simulink model "reverserotor"  (Simulink 10.0)
settings: Solver=ode23t  StartTime=0.0  StopTime=2  RelTol=1e-3  EnableMultiTasking=on
settings Model: Creator=lenovo  LastModifiedBy=asuresh4
settings DataIOCC: LimitDataPoints=on  SignalLoggingSaveFormat=ModelDataLogs
settings OptimizationCC: ExpressionDepthLimit=2147483647
settings DebuggingCC: SolverPrmCheckMsg=warning  FcnCallInpInsideContextMsg=warning  StateNameClashWarn=warning
settings ConfigComp: CovExternalEMLEnable=off

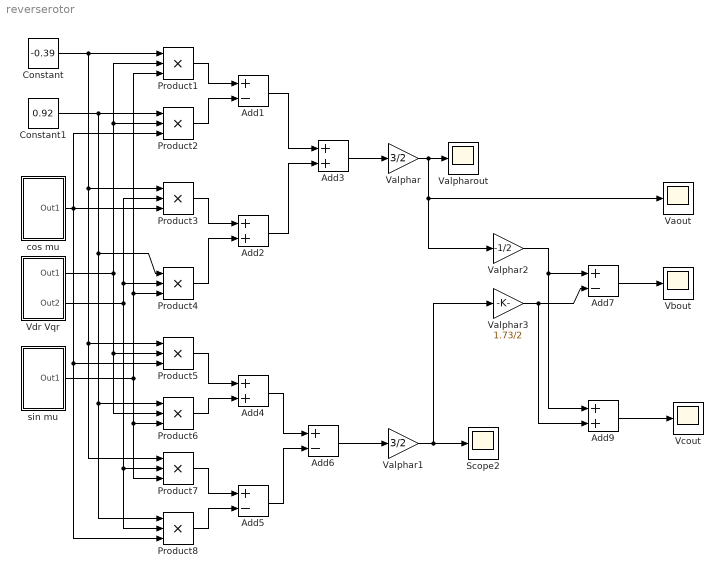
== system reverserotor ==
  Add{1,5..7} (4 alike) : Sum  Inputs=+-
  Add{2..4,9} (4 alike) : Sum
  Constant : Constant  Value=-0.39
  Constant1 : Constant  Value=0.92
  Product{1..8} (8 alike) : Product  Inputs=3  RndMeth=Zero
  Scope2 : Scope
  Valphar : Gain  Gain=3/2
  Valphar1 : Gain  Gain=3/2
  Valphar2 : Gain  Gain=-1/2
  Valphar3 : Gain  Gain=1.73/2
  Valpharout : Scope
  Vaout : Scope
  Vbout : Scope
  Vcout : Scope
  Vdr Vqr : Subsystem
  cos mu : Subsystem
  sin mu : Subsystem
  wires:
  Constant/1 -> Product1/1, Product3/1, Product5/1, Product7/1
  Vdr Vqr/1(Out1) -> Product1/2, Product2/2, Product5/2, Product6/2
  sin mu/1(Out1) -> Product1/3, Product4/3, Product6/3, Product7/3
  Constant1/1 -> Product2/1, Product4/1, Product6/1, Product8/1
  cos mu/1(Out1) -> Product3/3, Product2/3, Product5/3, Product8/3
  Product1/1 -> Add1/1
  Product2/1 -> Add1/2
  Vdr Vqr/2(Out2) -> Product3/2, Product4/2, Product7/2, Product8/2
  Product3/1 -> Add2/1
  Product4/1 -> Add2/2
  Add1/1 -> Add3/1
  Add2/1 -> Add3/2
  Add3/1 -> Valphar/1
  Valphar/1 -> Vaout/1, Valphar2/1, Valpharout/1
  Valphar1/1 -> Scope2/1, Valphar3/1
  Add6/1 -> Valphar1/1
  Add4/1 -> Add6/1
  Add5/1 -> Add6/2
  Product5/1 -> Add4/1
  Product6/1 -> Add4/2
  Product7/1 -> Add5/1
  Product8/1 -> Add5/2
  Add7/1 -> Vbout/1
  Valphar3/1 -> Add7/2, Add9/2
  Valphar2/1 -> Add7/1, Add9/1
  Add9/1 -> Vcout/1

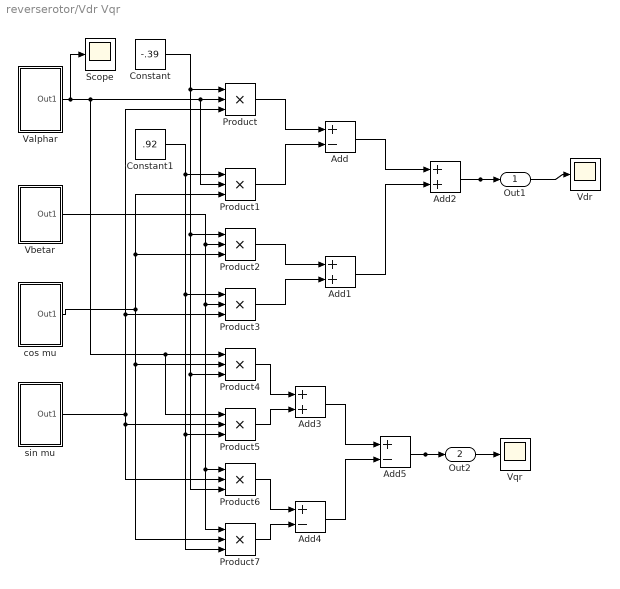
== system reverserotor/Vdr Vqr ==
  Add : Sum  Inputs=+-
  Add1 : Sum
  Add2 : Sum
  Add3 : Sum
  Add4 : Sum  Inputs=+-
  Add5 : Sum  Inputs=+-
  Constant : Constant  Value=-.39
  Constant1 : Constant  Value=.92
  Product{,1..7} (8 alike) : Product  Inputs=3  RndMeth=Zero
  Scope : Scope
  Valphar : Subsystem
  Vbetar : Subsystem
  Vdr : Scope
  Vqr : Scope
  cos mu : Subsystem
  sin mu : Subsystem
  Out1 : Outport
  Out2 : Outport  Port=2
  wires:
  Constant/1 -> Product/1, Product2/1, Product4/3, Product6/3
  sin mu/1(Out1) -> Product/3, Product3/3, Product5/2, Product6/2
  Valphar/1(Out1) -> Product/2, Product1/2, Product4/1, Product5/1, Scope/1
  Constant1/1 -> Product1/1, Product3/1, Product5/3, Product7/3
  cos mu/1(Out1) -> Product1/3, Product2/3, Product4/2, Product7/2
  Product/1 -> Add/1
  Product1/1 -> Add/2
  Vbetar/1(Out1) -> Product2/2, Product3/2, Product6/1, Product7/1
  Product2/1 -> Add1/1
  Product3/1 -> Add1/2
  Add/1 -> Add2/1
  Add1/1 -> Add2/2
  Add2/1 -> Vdr/1, Out1/1
  Product4/1 -> Add3/1
  Product5/1 -> Add3/2
  Product6/1 -> Add4/1
  Product7/1 -> Add4/2
  Add3/1 -> Add5/1
  Add4/1 -> Add5/2
  Add5/1 -> Vqr/1, Out2/1

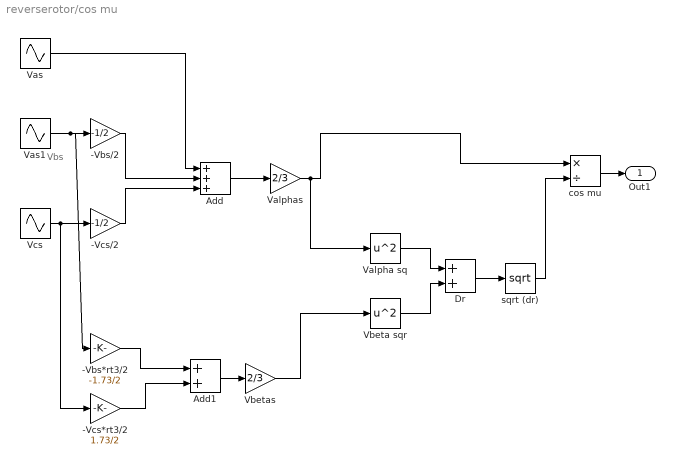
== system reverserotor/cos mu ==
  note: Vbs
  -Vbs*rt3/2 : Gain  Gain=-1.73/2
  -Vbs/2 : Gain  Gain=-1/2
  -Vcs*rt3/2 : Gain  Gain=1.73/2
  -Vcs/2 : Gain  Gain=-1/2
  Add : Sum  Inputs=+++
  Add1 : Sum
  Dr : Sum
  Valpha sq : Math  Operator=square  SaturateOnIntegerOverflow=on
  Valphas : Gain  Gain=2/3
  Vas : Sin  Amplitude=230  Frequency=314  SampleTime=0
  Vas1 : Sin  Amplitude=230  Frequency=314  Phase=-2.09  SampleTime=0
  Vbeta sqr : Math  Operator=square  SaturateOnIntegerOverflow=on
  Vbetas : Gain  Gain=2/3
  Vcs : Sin  Amplitude=230  Frequency=314  Phase=-4.18  SampleTime=0
  cos mu : Product  Inputs=*/
  sqrt (dr) : Math  Operator=sqrt  SaturateOnIntegerOverflow=on
  Out1 : Outport
  wires:
  Vas1/1 -> -Vbs/2/1, -Vbs*rt3/2/1
  Vcs/1 -> -Vcs/2/1, -Vcs*rt3/2/1
  Vas/1 -> Add/1
  -Vbs/2/1 -> Add/2
  -Vcs/2/1 -> Add/3
  Add/1 -> Valphas/1
  -Vbs*rt3/2/1 -> Add1/1
  -Vcs*rt3/2/1 -> Add1/2
  Add1/1 -> Vbetas/1
  Valphas/1 -> Valpha sq/1, cos mu/1
  Vbetas/1 -> Vbeta sqr/1
  Valpha sq/1 -> Dr/1
  Vbeta sqr/1 -> Dr/2
  Dr/1 -> sqrt (dr)/1
  sqrt (dr)/1 -> cos mu/2
  cos mu/1 -> Out1/1

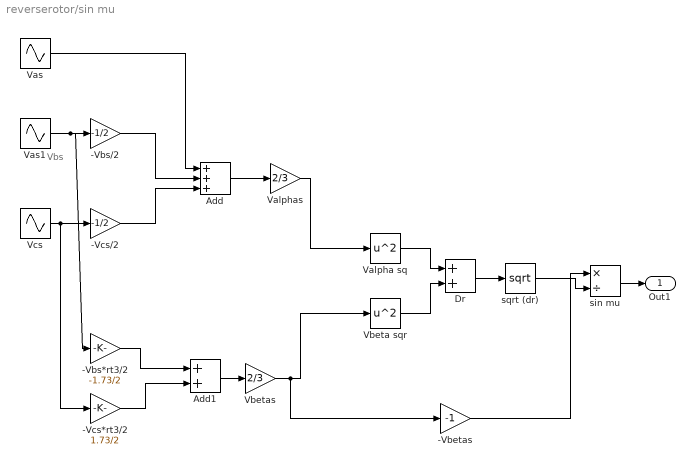
== system reverserotor/sin mu ==
  note: Vbs
  "-Vbetas " : Gain  Gain=-1
  -Vbs*rt3/2 : Gain  Gain=-1.73/2
  -Vbs/2 : Gain  Gain=-1/2
  -Vcs*rt3/2 : Gain  Gain=1.73/2
  -Vcs/2 : Gain  Gain=-1/2
  Add : Sum  Inputs=+++
  Add1 : Sum
  Dr : Sum
  Valpha sq : Math  Operator=square  SaturateOnIntegerOverflow=on
  Valphas : Gain  Gain=2/3
  Vas : Sin  Amplitude=230  Frequency=314  SampleTime=0
  Vas1 : Sin  Amplitude=230  Frequency=314  Phase=-2.09  SampleTime=0
  Vbeta sqr : Math  Operator=square  SaturateOnIntegerOverflow=on
  Vbetas : Gain  Gain=2/3
  Vcs : Sin  Amplitude=230  Frequency=314  Phase=-4.18  SampleTime=0
  sin mu : Product  Inputs=*/
  sqrt (dr) : Math  Operator=sqrt  SaturateOnIntegerOverflow=on
  Out1 : Outport
  wires:
  Vas1/1 -> -Vbs/2/1, -Vbs*rt3/2/1
  Vcs/1 -> -Vcs/2/1, -Vcs*rt3/2/1
  Vas/1 -> Add/1
  -Vbs/2/1 -> Add/2
  -Vcs/2/1 -> Add/3
  Add/1 -> Valphas/1
  -Vbs*rt3/2/1 -> Add1/1
  -Vcs*rt3/2/1 -> Add1/2
  Add1/1 -> Vbetas/1
  Valphas/1 -> Valpha sq/1
  Vbetas/1 -> "-Vbetas "/1, Vbeta sqr/1
  Valpha sq/1 -> Dr/1
  Vbeta sqr/1 -> Dr/2
  Dr/1 -> sqrt (dr)/1
  "-Vbetas "/1 -> sin mu/1
  sqrt (dr)/1 -> sin mu/2
  sin mu/1 -> Out1/1

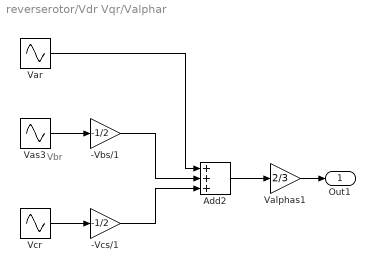
== system reverserotor/Vdr Vqr/Valphar ==
  note: Vbr
  -Vbs/1 : Gain  Gain=-1/2
  -Vcs/1 : Gain  Gain=-1/2
  Add2 : Sum  Inputs=+++
  Valphas1 : Gain  Gain=2/3
  Var : Sin  Amplitude=69  Frequency=314  SampleTime=0
  Vas3 : Sin  Amplitude=69  Frequency=314  Phase=-2.09  SampleTime=0
  Vcr : Sin  Amplitude=69  Frequency=314  Phase=-4.18  SampleTime=0
  Out1 : Outport
  wires:
  Vas3/1 -> -Vbs/1/1
  Vcr/1 -> -Vcs/1/1
  Var/1 -> Add2/1
  -Vbs/1/1 -> Add2/2
  -Vcs/1/1 -> Add2/3
  Add2/1 -> Valphas1/1
  Valphas1/1 -> Out1/1

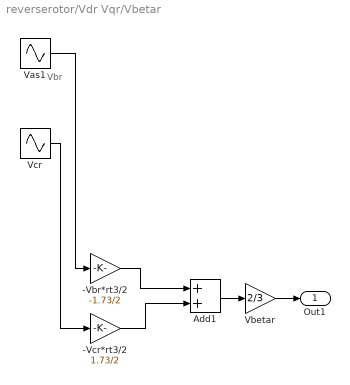
== system reverserotor/Vdr Vqr/Vbetar ==
  note: Vbr
  -Vbr*rt3/2 : Gain  Gain=-1.73/2
  -Vcr*rt3/2 : Gain  Gain=1.73/2
  Add1 : Sum
  Vas1 : Sin  Amplitude=69  Frequency=314  Phase=-2.09  SampleTime=0
  Vbetar : Gain  Gain=2/3
  Vcr : Sin  Amplitude=69  Frequency=314  Phase=-4.18  SampleTime=0
  Out1 : Outport
  wires:
  Vas1/1 -> -Vbr*rt3/2/1
  Vcr/1 -> -Vcr*rt3/2/1
  -Vbr*rt3/2/1 -> Add1/1
  -Vcr*rt3/2/1 -> Add1/2
  Add1/1 -> Vbetar/1
  Vbetar/1 -> Out1/1

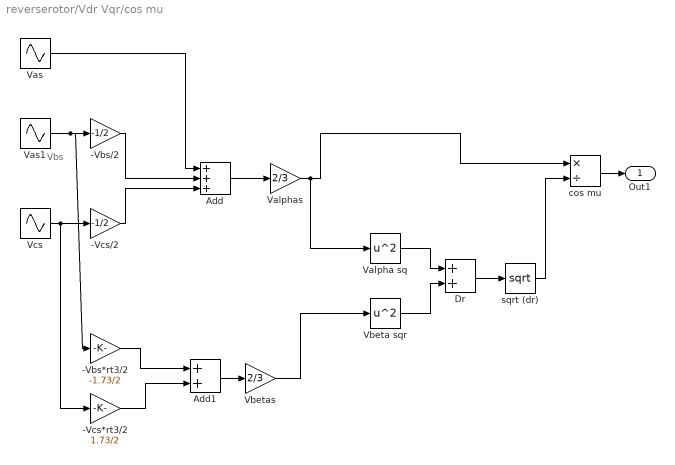
== system reverserotor/Vdr Vqr/cos mu ==
  note: Vbs
  -Vbs*rt3/2 : Gain  Gain=-1.73/2
  -Vbs/2 : Gain  Gain=-1/2
  -Vcs*rt3/2 : Gain  Gain=1.73/2
  -Vcs/2 : Gain  Gain=-1/2
  Add : Sum  Inputs=+++
  Add1 : Sum
  Dr : Sum
  Valpha sq : Math  Operator=square  SaturateOnIntegerOverflow=on
  Valphas : Gain  Gain=2/3
  Vas : Sin  Amplitude=230  Frequency=314  SampleTime=0
  Vas1 : Sin  Amplitude=230  Frequency=314  Phase=-2.09  SampleTime=0
  Vbeta sqr : Math  Operator=square  SaturateOnIntegerOverflow=on
  Vbetas : Gain  Gain=2/3
  Vcs : Sin  Amplitude=230  Frequency=314  Phase=-4.18  SampleTime=0
  cos mu : Product  Inputs=*/
  sqrt (dr) : Math  Operator=sqrt  SaturateOnIntegerOverflow=on
  Out1 : Outport
  wires:
  Vas1/1 -> -Vbs/2/1, -Vbs*rt3/2/1
  Vcs/1 -> -Vcs/2/1, -Vcs*rt3/2/1
  Vas/1 -> Add/1
  -Vbs/2/1 -> Add/2
  -Vcs/2/1 -> Add/3
  Add/1 -> Valphas/1
  -Vbs*rt3/2/1 -> Add1/1
  -Vcs*rt3/2/1 -> Add1/2
  Add1/1 -> Vbetas/1
  Valphas/1 -> Valpha sq/1, cos mu/1
  Vbetas/1 -> Vbeta sqr/1
  Valpha sq/1 -> Dr/1
  Vbeta sqr/1 -> Dr/2
  Dr/1 -> sqrt (dr)/1
  sqrt (dr)/1 -> cos mu/2
  cos mu/1 -> Out1/1

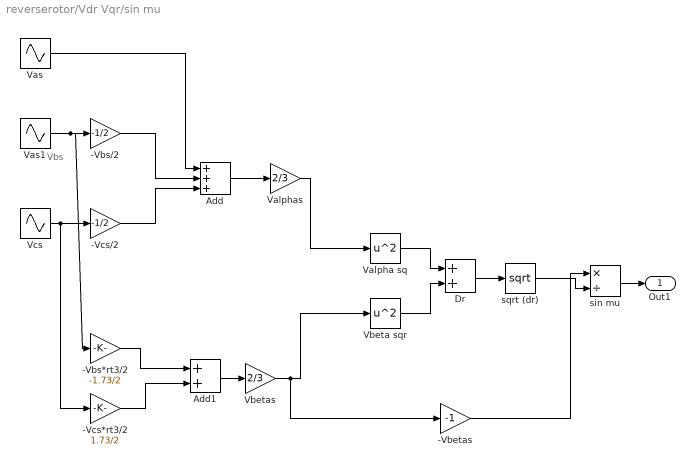
== system reverserotor/Vdr Vqr/sin mu ==
  note: Vbs
  "-Vbetas " : Gain  Gain=-1
  -Vbs*rt3/2 : Gain  Gain=-1.73/2
  -Vbs/2 : Gain  Gain=-1/2
  -Vcs*rt3/2 : Gain  Gain=1.73/2
  -Vcs/2 : Gain  Gain=-1/2
  Add : Sum  Inputs=+++
  Add1 : Sum
  Dr : Sum
  Valpha sq : Math  Operator=square  SaturateOnIntegerOverflow=on
  Valphas : Gain  Gain=2/3
  Vas : Sin  Amplitude=230  Frequency=314  SampleTime=0
  Vas1 : Sin  Amplitude=230  Frequency=314  Phase=-2.09  SampleTime=0
  Vbeta sqr : Math  Operator=square  SaturateOnIntegerOverflow=on
  Vbetas : Gain  Gain=2/3
  Vcs : Sin  Amplitude=230  Frequency=314  Phase=-4.18  SampleTime=0
  sin mu : Product  Inputs=*/
  sqrt (dr) : Math  Operator=sqrt  SaturateOnIntegerOverflow=on
  Out1 : Outport
  wires:
  Vas1/1 -> -Vbs/2/1, -Vbs*rt3/2/1
  Vcs/1 -> -Vcs/2/1, -Vcs*rt3/2/1
  Vas/1 -> Add/1
  -Vbs/2/1 -> Add/2
  -Vcs/2/1 -> Add/3
  Add/1 -> Valphas/1
  -Vbs*rt3/2/1 -> Add1/1
  -Vcs*rt3/2/1 -> Add1/2
  Add1/1 -> Vbetas/1
  Valphas/1 -> Valpha sq/1
  Vbetas/1 -> "-Vbetas "/1, Vbeta sqr/1
  Valpha sq/1 -> Dr/1
  Vbeta sqr/1 -> Dr/2
  Dr/1 -> sqrt (dr)/1
  "-Vbetas "/1 -> sin mu/1
  sqrt (dr)/1 -> sin mu/2
  sin mu/1 -> Out1/1
